simulink model "Test_ROS"  (R2019a)
settings: Solver=FixedStepAuto  StartTime=0.0  StopTime=inf  FixedStep=0.02  RelTol=1e-3
libraries: robotlib x2
settings Model: Creator=huic  LastModifiedBy=huic

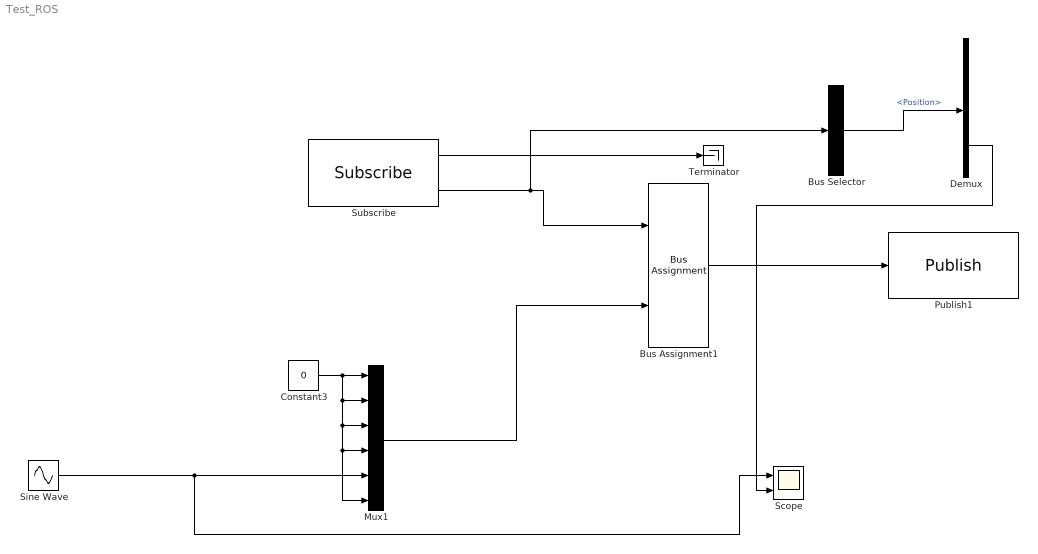
== system Test_ROS ==
  Bus Assignment1 : BusAssignment  AssignedSignals=Position
  Bus Selector : BusSelector  OutputSignals=Position
  Constant3 : Constant  Value=0
  Demux : Demux  Outputs=6
  Mux1 : Mux  Inputs=6
  Publish1 : robotlib/Publish  topicSource=Select from ROS network  topic=/joint_states  messageType=sensor_msgs/JointState  messageQueueLength=1
      settings: SourceProductBaseCode=RO
  Scope : Scope  NumInputPorts=2
  Sine Wave : Sin  Amplitude=1.57  Frequency=0.05  SampleTime=0
  Subscribe : robotlib/Subscribe  topicSource=Select from ROS network  topic=/joint_posStates  messageType=sensor_msgs/JointState  sampleTime=-1  messageQueueLength=1
      settings: SourceProductBaseCode=RO
  Terminator : Terminator
  wires:
  Subscribe/1 -> Terminator/1
  Subscribe/2 -> Bus Selector/1, Bus Assignment1/1
  Constant3/1 -> Mux1/6, Mux1/4, Mux1/3, Mux1/2, Mux1/1
  Mux1/1 -> Bus Assignment1/2
  Bus Assignment1/1 -> Publish1/1
  Bus Selector/1 -> Demux/1  "<Position>"
  Sine Wave/1 -> Mux1/5, Scope/1
  Demux/5 -> Scope/2
